simulink model "dc_motor_modelling"  (R2014b)
settings: Solver=ode23tb  StartTime=0.0  StopTime=10.0  RelTol=1e-3
settings Model: Creator=Amr Saleh  LastModifiedBy=Amr Saleh

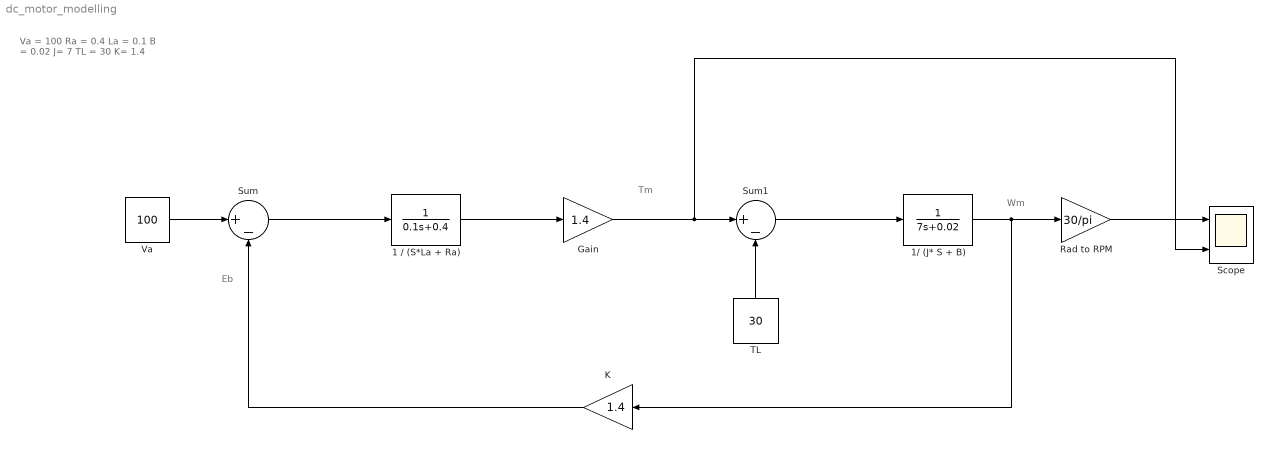
== system dc_motor_modelling ==
  note: Wm
  note: Tm
  note: Va = 100
      | Ra = 0.4
      | La = 0.1
      | B = 0.02
      | J= 7
      | TL = 30
      | K= 1.4
  note: Eb
  1 / (S*La + Ra) : TransferFcn  Denominator=[0.1 0.4]
  1/ (J* S + B) : TransferFcn  Denominator=[7 0.02]
  Gain : Gain  Gain=1.4
  K : Gain  Gain=1.4
  Rad to RPM : Gain  Gain=30/pi
  Scope : Scope  NumInputPorts=2
      settings: YMin=-5~-5  YMax=5~5
  Sum : Sum  Inputs=|+-
  Sum1 : Sum  Inputs=|+-
  TL : Constant  Value=30
  Va : Constant  Value=100
  wires:
  Va/1 -> Sum/1
  Sum/1 -> 1 / (S*La + Ra)/1
  1 / (S*La + Ra)/1 -> Gain/1
  Gain/1 -> Scope/2, Sum1/1
  Sum1/1 -> 1/ (J* S + B)/1
  1/ (J* S + B)/1 -> K/1, Rad to RPM/1
  Rad to RPM/1 -> Scope/1
  K/1 -> Sum/2
  TL/1 -> Sum1/2
